simulink model "subsystem"  (R2016b)
settings: Solver=FixedStepDiscrete  StartTime=0.0  StopTime=10.0  RelTol=1e-3
libraries: simulink x8
settings Model: Creator=Radwa  LastModifiedBy=Radwa
settings SolverCC: EnableConcurrentExecution=on
settings DataIOCC: ReturnWorkspaceOutputs=on
settings OptimizationCC: DefaultParameterBehavior=Inlined  EnhancedBackFolding=on  PassReuseOutputArgsAs=Individual arguments
settings DebuggingCC: ParameterTunabilityLossMsg=error
settings SFSimCC: SimUseLocalCustomCode=on
settings RTWCC: SystemTargetFile=ert.tlc  GenCodeOnly=on  TemplateMakefile=ert_default_tmf  Description=Embedded Coder  GenerateReport=on  RTWUseLocalCustomCode=on  IncludeHyperlinkInReport=on  LaunchReport=on  GenerateTraceInfo=on  GenerateTraceReport=on  GenerateTraceReportSl=on  GenerateTraceReportSf=on  GenerateTraceReportEml=on
settings CodeAppCC: ForceParamTrailComments=on  IgnoreCustomStorageClasses=off  OperatorAnnotations=on  SimulinkDataObjDesc=on  SFDataObjDesc=on  InsertBlockDesc=on
settings ERTTargetCC: TargetLangStandard=C99 (ISO)  MultiwordLength=256  GenerateSampleERTMain=on  InlinedParameterPlacement=NonHierarchical  ERTCustomFileTemplate=example_file_process.tlc

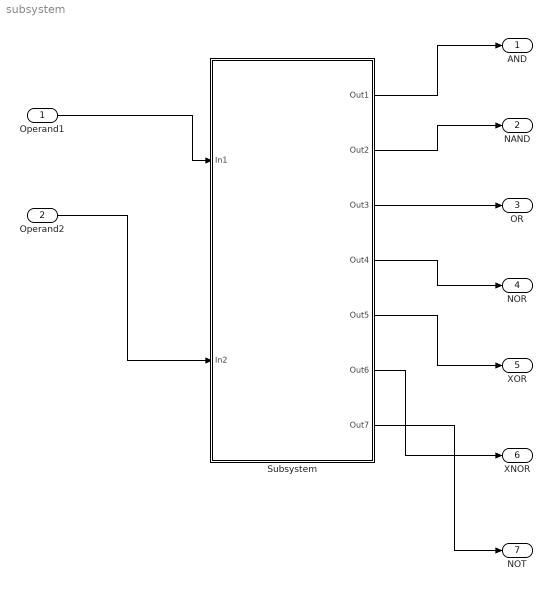
== system subsystem ==
  Operand1 : Inport  OutDataTypeStr=uint8
  Operand2 : Inport  Port=2  OutDataTypeStr=uint8
  Subsystem : Subsystem
  AND : Outport  OutDataTypeStr=uint8
  NAND : Outport  Port=2  OutDataTypeStr=uint8
  OR : Outport  Port=3  OutDataTypeStr=uint8
  NOR : Outport  Port=4  OutDataTypeStr=uint8
  XOR : Outport  Port=5  OutDataTypeStr=uint8
  XNOR : Outport  Port=6  OutDataTypeStr=uint8
  NOT : Outport  Port=7  OutDataTypeStr=uint8
  wires:
  Operand1/1 -> Subsystem/1(In1)
  Operand2/1 -> Subsystem/2(In2)
  Subsystem/1(Out1) -> AND/1
  Subsystem/2(Out2) -> NAND/1
  Subsystem/3(Out3) -> OR/1
  Subsystem/4(Out4) -> NOR/1
  Subsystem/5(Out5) -> XOR/1
  Subsystem/6(Out6) -> XNOR/1
  Subsystem/7(Out7) -> NOT/1

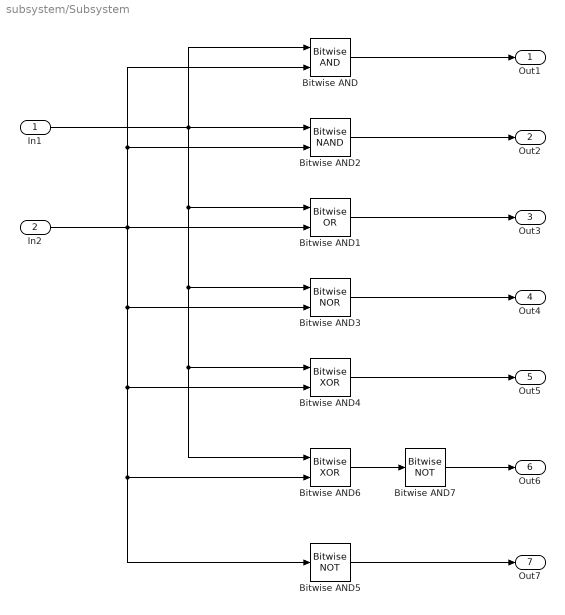
== system subsystem/Subsystem ==
  In1 : Inport
  In2 : Inport  Port=2
  Bitwise AND : simulink/Logic and Bit Operations/Bitwise Operator  logicop=AND  UseBitMask=off  NumInputPorts=2  BitMask=bin2dec('11011001')  BitMaskRealWorld=Stored Integer
  Bitwise AND1 : simulink/Logic and Bit Operations/Bitwise Operator  logicop=OR  UseBitMask=off  NumInputPorts=2  BitMask=bin2dec('11011001')  BitMaskRealWorld=Stored Integer
  Bitwise AND2 : simulink/Logic and Bit Operations/Bitwise Operator  logicop=NAND  UseBitMask=off  NumInputPorts=2  BitMask=bin2dec('11011001')  BitMaskRealWorld=Stored Integer
  Bitwise AND3 : simulink/Logic and Bit Operations/Bitwise Operator  logicop=NOR  UseBitMask=off  NumInputPorts=2  BitMask=bin2dec('11011001')  BitMaskRealWorld=Stored Integer
  Bitwise AND4 : simulink/Logic and Bit Operations/Bitwise Operator  logicop=XOR  UseBitMask=off  NumInputPorts=2  BitMask=bin2dec('11011001')  BitMaskRealWorld=Stored Integer
  Bitwise AND5 : simulink/Logic and Bit Operations/Bitwise Operator  logicop=NOT  UseBitMask=off  BitMask=bin2dec('11011001')  BitMaskRealWorld=Stored Integer
  Bitwise AND6 : simulink/Logic and Bit Operations/Bitwise Operator  logicop=XOR  UseBitMask=off  NumInputPorts=2  BitMask=bin2dec('11011001')  BitMaskRealWorld=Stored Integer
  Bitwise AND7 : simulink/Logic and Bit Operations/Bitwise Operator  logicop=NOT  UseBitMask=off  BitMask=bin2dec('11011001')  BitMaskRealWorld=Stored Integer
  Out1 : Outport
  Out2 : Outport  Port=2
  Out3 : Outport  Port=3
  Out4 : Outport  Port=4
  Out5 : Outport  Port=5
  Out6 : Outport  Port=6
  Out7 : Outport  Port=7
  wires:
  Bitwise AND4/1 -> Out5/1
  Bitwise AND6/1 -> Bitwise AND7/1
  Bitwise AND7/1 -> Out6/1
  Bitwise AND/1 -> Out1/1
  Bitwise AND3/1 -> Out4/1
  In2/1 -> Bitwise AND/2, Bitwise AND2/2, Bitwise AND1/2, Bitwise AND3/2, Bitwise AND4/2, Bitwise AND6/2, Bitwise AND5/1
  Bitwise AND2/1 -> Out2/1
  In1/1 -> Bitwise AND/1, Bitwise AND2/1, Bitwise AND6/1, Bitwise AND4/1, Bitwise AND3/1, Bitwise AND1/1
  Bitwise AND1/1 -> Out3/1
  Bitwise AND5/1 -> Out7/1
